simulink model "ADAS_AEB"  (R2026a)
settings: Solver=VariableStepAuto  StopTime=20
libraries: simulink x1
settings Model: Creator=nivru  LastModifiedBy=Pai

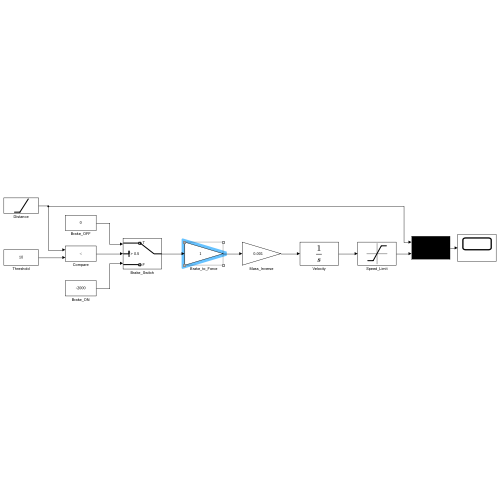
[thumbnail: Simulink's stored preview of the top-level diagram]
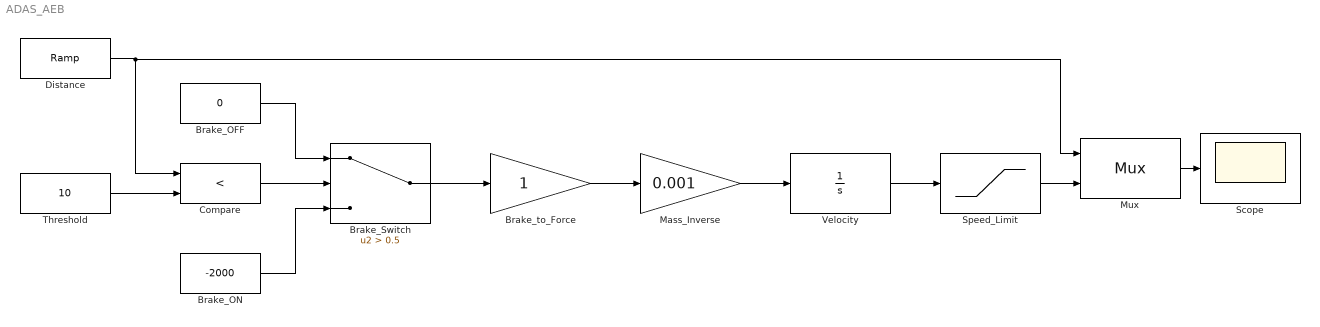
== system ADAS_AEB ==
  Brake_OFF : Constant  Value=0
  Brake_ON : Constant  Value=-2000
  Brake_Switch : Switch  Criteria=u2 > Threshold  Threshold=0.5  SaturateOnIntegerOverflow=off  InputSameDT=off
  Brake_to_Force : Gain
  Compare : RelationalOperator  Operator=<  OutDataTypeStr=boolean  RndMeth=Simplest  InputSameDT=off
  Distance : simulink/Sources/Ramp  slope=-5  start=5  InitialOutput=0
  Mass_Inverse : Gain  Gain=0.001
  Mux : Mux  Inputs=2
  Scope : Scope
      settings: ActiveDisplayYMinimum=-84.4375  ActiveDisplayYMaximum=9.9374999999999982
  Speed_Limit : Saturate  LowerLimit=0
  Threshold : Constant  Value=10
  Velocity : Integrator  InitialCondition=20
  wires:
  Distance/1 -> Compare/1, Mux/1
  Threshold/1 -> Compare/2
  Compare/1 -> Brake_Switch/2
  Brake_OFF/1 -> Brake_Switch/1
  Brake_ON/1 -> Brake_Switch/3
  Brake_Switch/1 -> Brake_to_Force/1
  Brake_to_Force/1 -> Mass_Inverse/1
  Mass_Inverse/1 -> Velocity/1
  Velocity/1 -> Speed_Limit/1
  Speed_Limit/1 -> Mux/2
  Mux/1 -> Scope/1
